simulink model "sldemo_househeat_non_linear"  (R2024b)
settings: Solver=ode45  StartTime=0.0  StopTime=2592000  FixedStep=1  RelTol=1e-3  AbsTol=1e-6
model workspace (MATLAB code in the model file):
  | % load initial conditions and physical properties from file
  | 
  | sldemo_househeat_data
values from neighbouring files (symbols this model uses):
  alpha = 0.01    [sldemo_househeat_data.m]
  cbrick = 850    [sldemo_househeat_data.m]
  cost = 0.25 / 3.6e6    (= 6.94444444444e-08)    [sldemo_househeat_data.m]
  epsilon = 0.9    [sldemo_househeat_data.m]
  Mbrick = 500 * wallArea    (= 100800)    [sldemo_househeat_data.m]
  QAerotermia = 14000    [sldemo_househeat_data.m]
  R0 = 1 / G_total    (= 0.0042955534856)    [sldemo_househeat_data.m]
  sigma = 5.670374419e-8    (= 5.670374419e-08)    [sldemo_househeat_data.m]
  TinIC = 20    [sldemo_househeat_data.m]
  wallArea = 2 * lenHouse * htHouse + 2 * widHouse * htHouse - windowArea    (= 201.6)    [sldemo_househeat_data.m]
undefined symbols (not defined in the file or in its folder): c, M, Mdot, THeater
Description:
  | Thermal Model of a House
  | 
  | This demo illustrates how you can use Simulink(R) to create the thermal model of
  | a house. This system models the outdoor environment, the thermal
  | characteristics of the house, and the house heating system.
  | 
  | The sldemo_househeat_data.m file initializes data in the model workspace.
  | To make changes, you can edit the model workspace directly or edit the MATLAB(R) file
  | and re-load the model workspace.
  | 
  | To view the model workspace, select View > Model Explorer
  | from the Simulink editor.
  | 
  | Note: Time is given in units of hours
settings Model: Creator=The MathWorks, Inc.  LastModifiedBy=fergusproctor
settings SolverCC: AutoScaleAbsTol=off  AlgebraicLoopSolver=TrustRegion
settings DataIOCC: ExternalInput=[]  InitialState=[]
settings OptimizationCC: BlockReduction=off  BooleanDataType=off  ReuseModelBlockBuffer=off  ExpressionDepthLimit=2147483647  InitFltsAndDblsToZero=on  LifeSpan=inf  BufferReusableBoundary=off
settings DebuggingCC: SaveWithParameterizedLinksMsg=none  UnderspecifiedInitializationDetection=Classic  MergeDetectMultiDrivingBlocksExec=none  SignalResolutionControl=TryResolveAllWithWarning  MultiTaskDSMMsg=warning  MultiTaskCondExecSysMsg=none  IntegerOverflowMsg=none  FcnCallInpInsideContextMsg=warning  UnconnectedInputMsg=warning  UnconnectedOutputMsg=warning  UnconnectedLineMsg=warning  BusObjectLabelMismatch=none  StateNameClashWarn=warning  SFUnexpectedBacktrackingDiag=warning  SFNoUnconditionalDefaultTransitionDiag=warning  SFExecutionAtInitializationDiag=none  IntegerSaturationMsg=none  ArithmeticOperatorsInVariantConditions=warning
settings HardwareCC: ProdBitPerPointer=32  ProdBitPerSizeT=32  ProdBitPerPtrDiffT=32  ProdLargestAtomicFloat=None  ProdIntDivRoundTo=Undefined  ProdEndianess=Unspecified  ProdWordSize=32  ProdHWDeviceType=32-bit Generic  TargetUnknown=on
settings ModelReferenceCC: EnableRefExpFcnMdlSchedulingChecks=on  PropagateSignalLabelsOutOfModel=off
settings SFSimCC: SimUseLocalCustomCode=off  CustomCodeUndefinedFunction=UseInterfaceOnly
settings RTWCC: RTWUseLocalCustomCode=off  GPUComputeCapability=3.5
settings CodeAppCC: StateflowObjectComments=on
settings GRTTargetCC: TargetFcnLib=ansi_tfl_tmw.mat  TargetLangStandard=C89/C90 (ANSI)  CombineOutputUpdateFcns=off  GRTInterface=on
settings ConfigComp: CovMetricSettings=dw  CovSaveCumulativeToWorkspaceVar=on  CovSaveSingleToWorkspaceVar=on  CovExternalEMLEnable=off

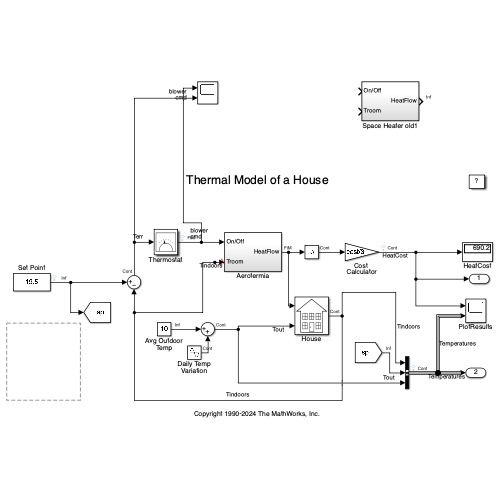
[thumbnail: Simulink's stored preview of the top-level diagram]
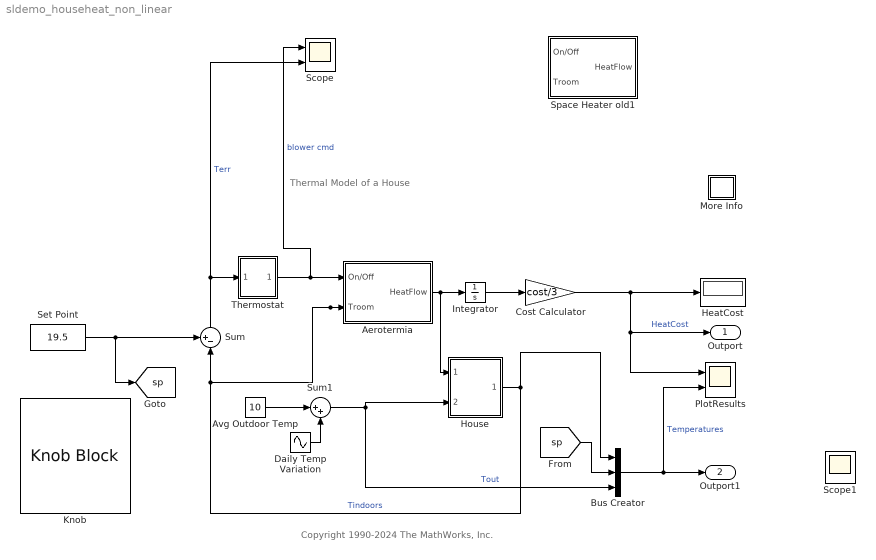
== system sldemo_househeat_non_linear ==
  note: Thermal Model of a House
  note: Copyright 1990-2024 The MathWorks, Inc.
  Aerotermia : Subsystem
  Avg Outdoor Temp : Constant  Value=10
  Bus Creator : BusCreator  Inputs=3
  Cost Calculator : Gain  Gain=cost/3  SaturateOnIntegerOverflow=on  OutDataTypeStr=Inherit: Same as input  ParamDataTypeStr=Inherit: Same as input
  Daily Temp Variation : Sin  Amplitude=7  Frequency=(2*pi)/(24*3600)  SampleTime=0
  HeatCost : Display
  House : Subsystem
      mask Display: image('HouseHeatHousePix.svg')
  Integrator : Integrator
  Knob : KnobBlock  ScaleMax=40
  More Info : Subsystem
      settings: OpenFcn=showExample('simulink_general/sldemo_househeatExample')
      mask Display: disp('?')
  PlotResults : Scope  NumInputPorts=2
  Scope : Scope  NumInputPorts=2
  Set Point : Constant  Value=19.5
  Space Heater old1 : Subsystem
  Sum : Sum  Inputs=+-|  InputSameDT=on  SaturateOnIntegerOverflow=on  OutDataTypeStr=Inherit: Same as first input
  Sum1 : Sum  Inputs=|++  InputSameDT=on  SaturateOnIntegerOverflow=on  OutDataTypeStr=Inherit: Same as first input
  Thermostat : Subsystem
      mask Display: image('HouseHeatThermostatPix.svg')
  Outport : Outport
  Outport1 : Outport  Port=2
  Scope1 : Scope
  tag scope: sp=global
  wires:
  Integrator/1 -> Cost Calculator/1
  Thermostat/1(Blower switch) -> Scope/1, Aerotermia/1(On/Off)  "blower cmd"
  Sum/1 -> Scope/2, Thermostat/1(Terr)  "Terr"
  Daily Temp Variation/1 -> Sum1/2
  Avg Outdoor Temp/1 -> Sum1/1
  House/1(Room Temp Troom) -> Bus Creator/1, Aerotermia/2(Troom), Sum/2  "Tindoors"
  Sum1/1 -> House/2(Outdoor Temp Tout), Bus Creator/3  "Tout"
  Aerotermia/1(HeatFlow) -> Integrator/1, House/1(Heater QDot In)
  Bus Creator/1 -> Outport1/1, PlotResults/2  "Temperatures"
  Cost Calculator/1 -> Outport/1, PlotResults/1, HeatCost/1  "HeatCost"
  Set Point/1 -> [sp], Sum/1
  [sp] -> Bus Creator/2

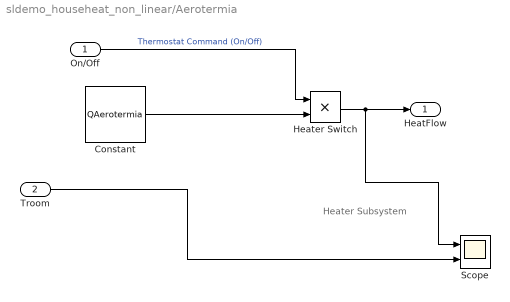
== system sldemo_househeat_non_linear/Aerotermia ==
  note: Heater Subsystem
  On/Off : Inport
  Troom : Inport  Port=2
  Constant : Constant  Value=QAerotermia
  Heater Switch : Product  RndMeth=Zero
  Scope : Scope  NumInputPorts=2
  HeatFlow : Outport  VectorParamsAs1DForOutWhenUnconnected=off
  wires:
  On/Off/1 -> Heater Switch/1  "Thermostat Command (On/Off)"
  Constant/1 -> Heater Switch/2
  Heater Switch/1 -> Scope/1, HeatFlow/1
  Troom/1 -> Scope/2

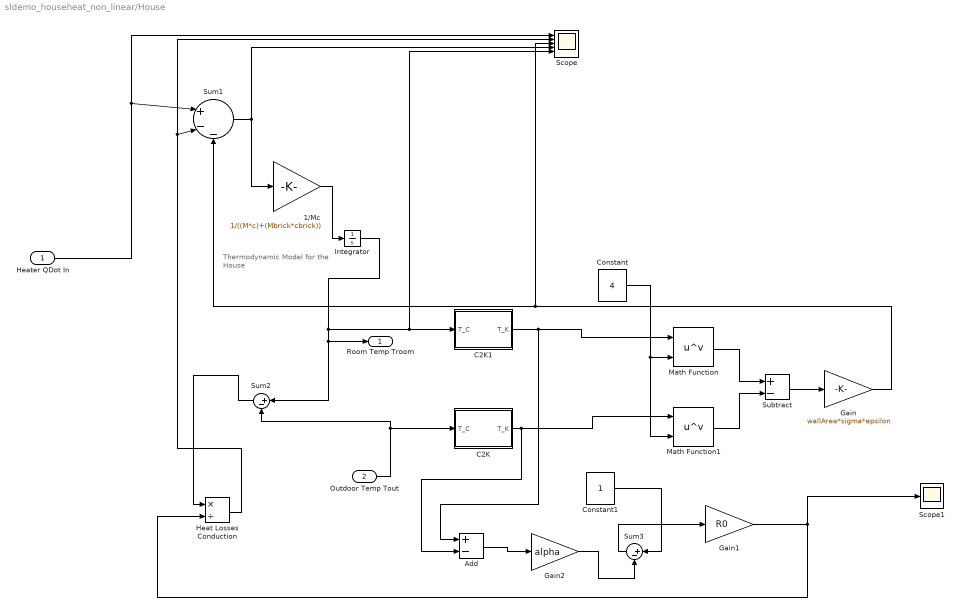
== system sldemo_househeat_non_linear/House ==
  note: Thermodynamic Model
      | for the House
  Heater QDot In : Inport
  Outdoor Temp Tout : Inport  Port=2
  1/Mc : Gain  Gain=1/((M*c)+(Mbrick*cbrick))  SaturateOnIntegerOverflow=on  OutDataTypeStr=Inherit: Same as input  ParamDataTypeStr=Inherit: Same as input
  Add : Sum  Inputs=+-
  C2K : MATLAB Function  TreatAsAtomicUnit=on
  C2K1 : MATLAB Function  TreatAsAtomicUnit=on
  Constant : Constant  Value=4
  Constant1 : Constant
  Gain : Gain  Gain=wallArea*sigma*epsilon
  Gain1 : Gain  Gain=R0
  Gain2 : Gain  Gain=alpha
  Heat Losses Conduction : Product  Inputs=*/
  Integrator : Integrator  InitialCondition=TinIC
  Math Function : Math  Operator=pow
  Math Function1 : Math  Operator=pow
  Scope : Scope  NumInputPorts=5
  Scope1 : Scope
  Subtract : Sum  Inputs=+-
  Sum1 : Sum  Inputs=|+--  InputSameDT=on  SaturateOnIntegerOverflow=on  OutDataTypeStr=Inherit: Same as first input
  Sum2 : Sum  Inputs=|+-  InputSameDT=on  SaturateOnIntegerOverflow=on  OutDataTypeStr=Inherit: Same as first input
  Sum3 : Sum  Inputs=|+-  InputSameDT=on  SaturateOnIntegerOverflow=on  OutDataTypeStr=Inherit: Same as first input
  Room Temp Troom : Outport  InitialOutput=0  VectorParamsAs1DForOutWhenUnconnected=off
  wires:
  Outdoor Temp Tout/1 -> Sum2/2, C2K/1(T_C)
  Heater QDot In/1 -> Scope/1, Sum1/1
  Sum1/1 -> 1/Mc/1, Scope/4
  Sum2/1 -> Heat Losses Conduction/1
  1/Mc/1 -> Integrator/1
  Integrator/1 -> Room Temp Troom/1, Sum2/1, Scope/5, C2K1/1(T_C)
  C2K1/1(T_K) -> Add/1, Math Function/1
  C2K/1(T_K) -> Add/2, Math Function1/1
  Constant/1 -> Math Function1/2, Math Function/2
  Math Function/1 -> Subtract/1
  Math Function1/1 -> Subtract/2
  Subtract/1 -> Gain/1
  Constant1/1 -> Sum3/1
  Gain2/1 -> Sum3/2
  Sum3/1 -> Gain1/1
  Add/1 -> Gain2/1
  Gain1/1 -> Heat Losses Conduction/2, Scope1/1
  Heat Losses Conduction/1 -> Scope/2, Sum1/2
  Gain/1 -> Scope/3, Sum1/3

== system sldemo_househeat_non_linear/More Info ==

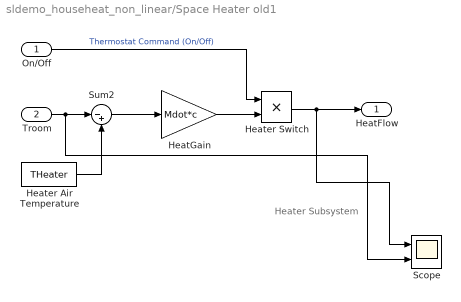
== system sldemo_househeat_non_linear/Space Heater old1 ==
  note: Heater Subsystem
  On/Off : Inport
  Troom : Inport  Port=2
  HeatGain : Gain  Gain=Mdot*c
  Heater Air Temperature : Constant  Value=THeater
  Heater Switch : Product  RndMeth=Zero
  Scope : Scope  NumInputPorts=2
  Sum2 : Sum  Inputs=|-+
  HeatFlow : Outport  VectorParamsAs1DForOutWhenUnconnected=off
  wires:
  Heater Air Temperature/1 -> Sum2/2
  Troom/1 -> Scope/2, Sum2/1
  Sum2/1 -> HeatGain/1
  On/Off/1 -> Heater Switch/1  "Thermostat Command (On/Off)"
  HeatGain/1 -> Heater Switch/2
  Heater Switch/1 -> Scope/1, HeatFlow/1

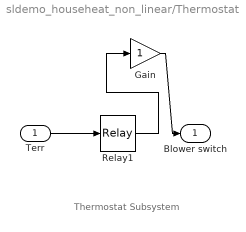
== system sldemo_househeat_non_linear/Thermostat ==
  note: Thermostat Subsystem
  Terr : Inport
  Gain : Gain
  Relay1 : Relay  OnSwitchValue=2  OffSwitchValue=-2
  Blower switch : Outport  InitialOutput=0  VectorParamsAs1DForOutWhenUnconnected=off
  wires:
  Terr/1 -> Relay1/1
  Relay1/1 -> Gain/1
  Gain/1 -> Blower switch/1

== matlab function sldemo_househeat_non_linear/House/C2K ==
  data: T_C input; T_K output



function T_K = celsiusToKelvin(T_C)
T_K = T_C + 273.15;
end

== matlab function sldemo_househeat_non_linear/House/C2K1 ==
  data: T_C input; T_K output



function T_K = celsiusToKelvin(T_C)
T_K = T_C + 273.15;
end
